simulink model "original_model"  (R2016b)
settings: Solver=FixedStepAuto  StartTime=0.0  StopTime=1  FixedStep=0.02  RelTol=1e-3
values from neighbouring files (symbols this model uses):
  rho = [rho1 rho2 rho3 rho4]    [leastSquare.m]    (also in leastSquare2.m = (transpose(A)*A)\transpose(A)*b; parameters.mat = [-1.71136748701 2.88809791639 8.34085809492 -3.97806529373])
  sig = (transpose(A)*A)\transpose(A)*b    [leastSquare.m]    (also in leastSquare2.m; parameters.mat = [11.0155519472 -6.53364462652 33.0155389324 0.441275229296 1)
settings Model: Creator=Ernie  LastModifiedBy=Ernie

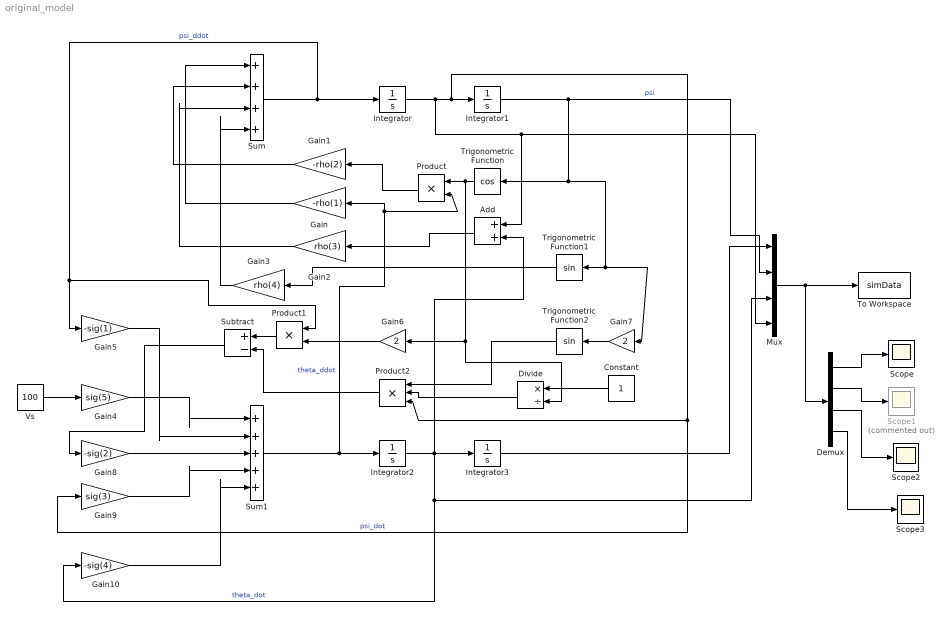
== system original_model ==
  Add : Sum
  Constant : Constant
  Demux : Demux
  Divide : Product  Inputs=*/
  Gain : Gain  Gain=-rho(1)
  Gain1 : Gain  Gain=-rho(2)
  Gain10 : Gain  Gain=-sig(4)
  Gain2 : Gain  Gain=rho(3)
  Gain3 : Gain  Gain=rho(4)
  Gain4 : Gain  Gain=sig(5)
  Gain5 : Gain  Gain=-sig(1)
  Gain6 : Gain  Gain=2
  Gain7 : Gain  Gain=2
  Gain8 : Gain  Gain=-sig(2)
  Gain9 : Gain  Gain=sig(3)
  Integrator{,1..3} (4 alike) : Integrator
  Mux : Mux
  Product : Product
  Product1 : Product
  Product2 : Product  Inputs=3
  Scope : Scope
  Scope1 : Scope  Commented=on
  Scope2 : Scope
  Scope3 : Scope
  Subtract : Sum  Inputs=+-
  Sum : Sum  Inputs=|++++|
  Sum1 : Sum  Inputs=|+++++|
  To Workspace : ToWorkspace  VariableName=simData  SaveFormat=Timeseries  SampleTime=-1
  Trigonometric Function : Trigonometry  Operator=cos
  Trigonometric Function1 : Trigonometry
  Trigonometric Function2 : Trigonometry
  Vs : Constant  Value=100
  wires:
  Integrator/1 -> Mux/4, Add/1, Integrator1/1, Gain9/1, Product2/3  "psi_dot"
  Integrator2/1 -> Mux/3, Gain10/1, Add/2, Integrator3/1  "theta_dot"
  Sum/1 -> Product1/1, Gain5/1, Integrator/1  "psi_ddot"
  Sum1/1 -> Product/2, Gain/1, Integrator2/1  "theta_ddot"
  Gain/1 -> Sum/1
  Integrator1/1 -> Mux/2, Gain7/1, Trigonometric Function1/1, Trigonometric Function/1  "psi"
  Trigonometric Function/1 -> Divide/2, Gain6/1, Product/1
  Product/1 -> Gain1/1
  Gain1/1 -> Sum/2
  Add/1 -> Gain2/1
  Gain2/1 -> Sum/3
  Trigonometric Function1/1 -> Gain3/1
  Gain3/1 -> Sum/4
  Vs/1 -> Gain4/1
  Gain4/1 -> Sum1/1
  Gain5/1 -> Sum1/2
  Gain6/1 -> Product1/2
  Product1/1 -> Subtract/1
  Gain7/1 -> Trigonometric Function2/1
  Trigonometric Function2/1 -> Product2/1
  Divide/1 -> Product2/2
  Product2/1 -> Subtract/2
  Constant/1 -> Divide/1
  Subtract/1 -> Gain8/1
  Gain8/1 -> Sum1/3
  Gain9/1 -> Sum1/4
  Gain10/1 -> Sum1/5
  Mux/1 -> Demux/1, To Workspace/1
  Integrator3/1 -> Mux/1
  Demux/2 -> Scope1/1
  Demux/1 -> Scope/1
  Demux/3 -> Scope2/1
  Demux/4 -> Scope3/1
